simulink model "integrator_ext_IC_vector_test_tmp"  (Simulink 8.3)
settings: Solver=ode45  StartTime=0.0  StopTime=10.0  RelTol=1e-3
undefined symbols (not defined in the file): DiscIntNeverNeededParam
settings Model: Creator=arnaud  LastModifiedBy=hbourbou
settings DataIOCC: SaveFormat=Structure
settings OptimizationCC: ExpressionDepthLimit=2147483647
settings DebuggingCC: FcnCallInpInsideContextMsg=EnableAllAsWarning  FrameProcessingCompatibilityMsg=error

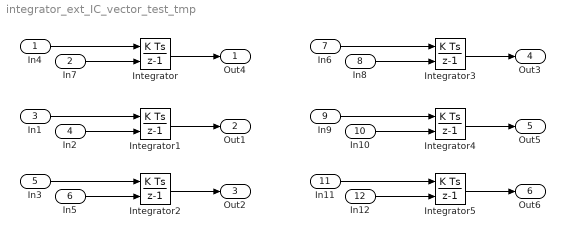
== system integrator_ext_IC_vector_test_tmp ==
  In4 : Inport  OutDataTypeStr=double  PortDimensions=3
  In7 : Inport  Port=2  OutDataTypeStr=double
  In1 : Inport  Port=3  OutDataTypeStr=double  PortDimensions=1
  In2 : Inport  Port=4  OutDataTypeStr=double  PortDimensions=3
  In3 : Inport  Port=5  OutDataTypeStr=double  PortDimensions=3
  In5 : Inport  Port=6  OutDataTypeStr=double  PortDimensions=3
  In6 : Inport  Port=7  OutDataTypeStr=double  PortDimensions=3
  In8 : Inport  Port=8  OutDataTypeStr=double
  In9 : Inport  Port=9  OutDataTypeStr=double  PortDimensions=1
  In10 : Inport  Port=10  OutDataTypeStr=double  PortDimensions=3
  In11 : Inport  Port=11  OutDataTypeStr=double  PortDimensions=3
  In12 : Inport  Port=12  OutDataTypeStr=double  PortDimensions=3
  Integrator : DiscreteIntegrator  InitialConditionSource=external  SampleTime=1.0  ICPrevOutput=DiscIntNeverNeededParam  ICPrevScaledInput=DiscIntNeverNeededParam  mask(DiscretizedDiscreteIntegrator){}
      mask init:
      | %zoh
  Integrator1 : DiscreteIntegrator  InitialConditionSource=external  SampleTime=1.0  ICPrevOutput=DiscIntNeverNeededParam  ICPrevScaledInput=DiscIntNeverNeededParam  mask(DiscretizedDiscreteIntegrator){}
      mask init:
      | %zoh
  Integrator2 : DiscreteIntegrator  InitialConditionSource=external  SampleTime=1.0  ICPrevOutput=DiscIntNeverNeededParam  ICPrevScaledInput=DiscIntNeverNeededParam  mask(DiscretizedDiscreteIntegrator){}
      mask init:
      | %zoh
  Integrator3 : DiscreteIntegrator  gainval=[2 5 .9]  InitialConditionSource=external  SampleTime=1.0  ICPrevOutput=DiscIntNeverNeededParam  ICPrevScaledInput=DiscIntNeverNeededParam  mask(DiscretizedDiscreteIntegrator){}
      mask init:
      | %zoh
  Integrator4 : DiscreteIntegrator  gainval=[2 5 .9]  InitialConditionSource=external  SampleTime=1.0  ICPrevOutput=DiscIntNeverNeededParam  ICPrevScaledInput=DiscIntNeverNeededParam  mask(DiscretizedDiscreteIntegrator){}
      mask init:
      | %zoh
  Integrator5 : DiscreteIntegrator  gainval=[2 5 .9]  InitialConditionSource=external  SampleTime=1.0  ICPrevOutput=DiscIntNeverNeededParam  ICPrevScaledInput=DiscIntNeverNeededParam  mask(DiscretizedDiscreteIntegrator){}
      mask init:
      | %zoh
  Out4 : Outport
  Out1 : Outport  Port=2
  Out2 : Outport  Port=3
  Out3 : Outport  Port=4
  Out5 : Outport  Port=5
  Out6 : Outport  Port=6
  wires:
  In4/1 -> Integrator/1
  Integrator/1 -> Out4/1
  In7/1 -> Integrator/2
  In1/1 -> Integrator1/1
  Integrator1/1 -> Out1/1
  In2/1 -> Integrator1/2
  In3/1 -> Integrator2/1
  Integrator2/1 -> Out2/1
  In5/1 -> Integrator2/2
  In6/1 -> Integrator3/1
  Integrator3/1 -> Out3/1
  In8/1 -> Integrator3/2
  In9/1 -> Integrator4/1
  Integrator4/1 -> Out5/1
  In10/1 -> Integrator4/2
  In11/1 -> Integrator5/1
  Integrator5/1 -> Out6/1
  In12/1 -> Integrator5/2
